simulink model "Suspension"  (R2019b)
settings: Solver=VariableStepAuto  StartTime=0.0  StopTime=10.0  RelTol=1e-3
values from neighbouring files (symbols this model uses):
  cfs = 1290    [Suspension_parameter.m]
  cft = 1000    [Suspension_parameter.m]
  crs = 1620    [Suspension_parameter.m]
  crt = 1000    [Suspension_parameter.m]
  iyy = 2460    [Suspension_parameter.m]
  kfs = 19960    [Suspension_parameter.m]
  kft = 175500    [Suspension_parameter.m]
  krs = 17500    [Suspension_parameter.m]
  krt = 175500    [Suspension_parameter.m]
  lf = 2.3    [Suspension_parameter.m]
  lr = 2.3    [Suspension_parameter.m]
  mc = 700    [Suspension_parameter.m]
  mf = 40    [Suspension_parameter.m]
  mr = 35.5    [Suspension_parameter.m]
libraries: simulink x4
(part 2 of 2)

== system Suspension/Sky Hook/Front Displacement(Zf)/Road condition 2  ==
  Product : Product  Inputs=3
  Saturation : Saturate  LowerLimit=0
  Scope : Scope
  Signal Generator : SignalGenerator  Amplitude=0.15  Frequency=1.852
  Step : Step  SampleTime=1.08
  Step1 : Step  Before=1  After=0  SampleTime=4
  Out2 : Outport
  wires:
  Signal Generator/1 -> Product/1
  Product/1 -> Out2/1, Saturation/1
  Step/1 -> Product/2
  Step1/1 -> Product/3
  Saturation/1 -> Scope/1

== system Suspension/Sky Hook/Front Displacement(Zf)/Sky Hook_f ==
  Zc_dot : Inport
  Zf_dot : Inport  Port=2
  Add : Sum  Inputs=+-
  Constant : Constant  Value=2838
  Constant1 : Constant  Value=258
  If : If  IfExpression=u1 >= 0  ZeroCross=off
  Merge : Merge
  Product : Product
  Switch Case Action Subsystem : Subsystem  TreatAsAtomicUnit=on
  Switch Case Action Subsystem1 : Subsystem  TreatAsAtomicUnit=on
  Out1 : Outport
  wires:
  Constant1/1 -> Switch Case Action Subsystem1/1(In1)
  Zc_dot/1 -> Product/1, Add/1
  Switch Case Action Subsystem/1(Out1) -> Merge/1
  Switch Case Action Subsystem1/1(Out1) -> Merge/2
  Add/1 -> Product/2
  Product/1 -> If/1
  If/2 -> Switch Case Action Subsystem1/Action
  If/1 -> Switch Case Action Subsystem/Action
  Constant/1 -> Switch Case Action Subsystem/1(In1)
  Zf_dot/1 -> Add/2
  Merge/1 -> Out1/1

== system Suspension/Sky Hook/Rear Displacement(Zr)/Road conditiion 1 ==
  Gain : Gain
  Product : Product  Inputs=3
  Scope : Scope
  Signal Generator : SignalGenerator  Amplitude=0.15  Frequency=1.852  Units=rad/sec
  Step : Step  SampleTime=1.08
  Step1 : Step  Before=1  After=0  SampleTime=1.35
  Out1 : Outport
  wires:
  Gain/1 -> Out1/1
  Step1/1 -> Product/3
  Product/1 -> Gain/1, Scope/1
  Step/1 -> Product/2
  Signal Generator/1 -> Product/1

== system Suspension/Sky Hook/Rear Displacement(Zr)/Road condition 2  ==
  Product : Product  Inputs=3
  Saturation : Saturate  LowerLimit=0
  Scope : Scope
  Signal Generator : SignalGenerator  Amplitude=0.15  Frequency=1.852
  Step : Step  SampleTime=1.08
  Step1 : Step  Before=1  After=0  SampleTime=4
  Out2 : Outport
  wires:
  Signal Generator/1 -> Product/1
  Product/1 -> Out2/1, Saturation/1
  Step/1 -> Product/2
  Step1/1 -> Product/3
  Saturation/1 -> Scope/1

== system Suspension/Sky Hook/Rear Displacement(Zr)/Sky Hook_r1 ==
  Zc_dot : Inport
  Zr_dot : Inport  Port=2
  Add : Sum  Inputs=+-
  Constant : Constant  Value=2838
  Constant1 : Constant  Value=258
  If : If  IfExpression=u1 >= 0  ZeroCross=off
  Merge : Merge
  Product : Product
  Switch Case Action Subsystem : Subsystem  TreatAsAtomicUnit=on
  Switch Case Action Subsystem1 : Subsystem  TreatAsAtomicUnit=on
  Out1 : Outport
  wires:
  Constant1/1 -> Switch Case Action Subsystem1/1(In1)
  Zc_dot/1 -> Product/1, Add/1
  Switch Case Action Subsystem/1(Out1) -> Merge/1
  Switch Case Action Subsystem1/1(Out1) -> Merge/2
  Add/1 -> Product/2
  Product/1 -> If/1
  If/2 -> Switch Case Action Subsystem1/Action
  If/1 -> Switch Case Action Subsystem/Action
  Constant/1 -> Switch Case Action Subsystem/1(In1)
  Zr_dot/1 -> Add/2
  Merge/1 -> Out1/1

== system Suspension/Ground Hook/Body Displacement(Zc)/Ground_hook_f/Switch Case Action Subsystem ==
  1 : Inport
  Action Port : ActionPort  ActionPortLabel=if(u1 >= 0)
  Csa : Outport
  wires:
  1/1 -> Csa/1

== system Suspension/Ground Hook/Body Displacement(Zc)/Ground_hook_f/Switch Case Action Subsystem2 ==
  In1 : Inport
  Action Port : ActionPort  ActionPortLabel=else
  Out1 : Outport
  wires:
  In1/1 -> Out1/1

== system Suspension/Ground Hook/Body Displacement(Zc)/Ground_hook_r/Switch Case Action Subsystem ==
  1 : Inport
  Action Port : ActionPort  ActionPortLabel=if(u1 >= 0)
  Csa : Outport
  wires:
  1/1 -> Csa/1

== system Suspension/Ground Hook/Body Displacement(Zc)/Ground_hook_r/Switch Case Action Subsystem2 ==
  In1 : Inport
  Action Port : ActionPort  ActionPortLabel=else
  Out1 : Outport
  wires:
  In1/1 -> Out1/1

== system Suspension/Ground Hook/Front Displacement(Zf)/Ground_hook_f/Switch Case Action Subsystem ==
  1 : Inport
  Action Port : ActionPort  ActionPortLabel=if(u1 >= 0)
  Csa : Outport
  wires:
  1/1 -> Csa/1

== system Suspension/Ground Hook/Front Displacement(Zf)/Ground_hook_f/Switch Case Action Subsystem2 ==
  In1 : Inport
  Action Port : ActionPort  ActionPortLabel=else
  Out1 : Outport
  wires:
  In1/1 -> Out1/1

== system Suspension/Ground Hook/Rear Displacement(Zr)/Ground_hook_r/Switch Case Action Subsystem ==
  1 : Inport
  Action Port : ActionPort  ActionPortLabel=if(u1 >= 0)
  Csa : Outport
  wires:
  1/1 -> Csa/1

== system Suspension/Ground Hook/Rear Displacement(Zr)/Ground_hook_r/Switch Case Action Subsystem2 ==
  In1 : Inport
  Action Port : ActionPort  ActionPortLabel=else
  Out1 : Outport
  wires:
  In1/1 -> Out1/1

== system Suspension/Hybird Hook/Body Displacement(Zc)/HybridHook_f/GroundHook ==
  In1 : Inport
  In2 : Inport  Port=2
  Add5 : Sum  Inputs=+-
  Constant : Constant  Value=2838
  Constant1 : Constant  Value=258
  Gain9 : Gain  Gain=-1
  If : If  IfExpression=u1 >= 0  ZeroCross=off
  Merge : Merge
  Product : Product
  Switch Case Action Subsystem : Subsystem  TreatAsAtomicUnit=on
  Switch Case Action Subsystem2 : Subsystem  TreatAsAtomicUnit=on
  Out1 : Outport
  wires:
  Gain9/1 -> Product/2
  In2/1 -> Gain9/1, Add5/2
  Product/1 -> If/1
  If/2 -> Switch Case Action Subsystem2/Action
  Switch Case Action Subsystem/1(Csa) -> Merge/1
  Switch Case Action Subsystem2/1(Out1) -> Merge/2
  Constant1/1 -> Switch Case Action Subsystem2/1(In1)
  If/1 -> Switch Case Action Subsystem/Action
  In1/1 -> Add5/1
  Constant/1 -> Switch Case Action Subsystem/1(1)
  Add5/1 -> Product/1
  Merge/1 -> Out1/1

== system Suspension/Hybird Hook/Body Displacement(Zc)/HybridHook_f/SkyHook ==
  In1 : Inport
  In2 : Inport  Port=2
  Add : Sum  Inputs=+-
  Constant2 : Constant  Value=2838
  Constant3 : Constant  Value=258
  If1 : If  IfExpression=u1 >= 0  ZeroCross=off
  Merge1 : Merge
  Product1 : Product
  Switch Case Action Subsystem1 : Subsystem  TreatAsAtomicUnit=on
  Switch Case Action Subsystem3 : Subsystem  TreatAsAtomicUnit=on
  Out1 : Outport
  wires:
  Product1/1 -> If1/1
  Constant2/1 -> Switch Case Action Subsystem1/1(In1)
  If1/1 -> Switch Case Action Subsystem1/Action
  Add/1 -> Product1/2
  Switch Case Action Subsystem1/1(Out1) -> Merge1/1
  Constant3/1 -> Switch Case Action Subsystem3/1(In1)
  In1/1 -> Product1/1, Add/1
  If1/2 -> Switch Case Action Subsystem3/Action
  Switch Case Action Subsystem3/1(Out1) -> Merge1/2
  Merge1/1 -> Out1/1
  In2/1 -> Add/2

== system Suspension/Hybird Hook/Body Displacement(Zc)/HybridHook_r/GroundHook ==
  In1 : Inport
  In2 : Inport  Port=2
  Add5 : Sum  Inputs=+-
  Constant : Constant  Value=2838
  Constant1 : Constant  Value=258
  Gain9 : Gain  Gain=-1
  If : If  IfExpression=u1 >= 0  ZeroCross=off
  Merge : Merge
  Product : Product
  Switch Case Action Subsystem : Subsystem  TreatAsAtomicUnit=on
  Switch Case Action Subsystem2 : Subsystem  TreatAsAtomicUnit=on
  Out1 : Outport
  wires:
  Gain9/1 -> Product/2
  In2/1 -> Gain9/1, Add5/2
  Product/1 -> If/1
  If/2 -> Switch Case Action Subsystem2/Action
  Switch Case Action Subsystem/1(Csa) -> Merge/1
  Switch Case Action Subsystem2/1(Out1) -> Merge/2
  Constant1/1 -> Switch Case Action Subsystem2/1(In1)
  If/1 -> Switch Case Action Subsystem/Action
  In1/1 -> Add5/1
  Constant/1 -> Switch Case Action Subsystem/1(1)
  Add5/1 -> Product/1
  Merge/1 -> Out1/1

== system Suspension/Hybird Hook/Body Displacement(Zc)/HybridHook_r/SkyHook ==
  In1 : Inport
  In2 : Inport  Port=2
  Add : Sum  Inputs=+-
  Constant2 : Constant  Value=2838
  Constant3 : Constant  Value=258
  If1 : If  IfExpression=u1 >= 0  ZeroCross=off
  Merge1 : Merge
  Product1 : Product
  Switch Case Action Subsystem1 : Subsystem  TreatAsAtomicUnit=on
  Switch Case Action Subsystem3 : Subsystem  TreatAsAtomicUnit=on
  Out1 : Outport
  wires:
  Product1/1 -> If1/1
  Constant2/1 -> Switch Case Action Subsystem1/1(In1)
  If1/1 -> Switch Case Action Subsystem1/Action
  Add/1 -> Product1/2
  Switch Case Action Subsystem1/1(Out1) -> Merge1/1
  Constant3/1 -> Switch Case Action Subsystem3/1(In1)
  In1/1 -> Product1/1, Add/1
  If1/2 -> Switch Case Action Subsystem3/Action
  Switch Case Action Subsystem3/1(Out1) -> Merge1/2
  Merge1/1 -> Out1/1
  In2/1 -> Add/2

== system Suspension/Hybird Hook/Front Displacement(Zf)/HybridHook_f/GroundHook ==
  In1 : Inport
  In2 : Inport  Port=2
  Add5 : Sum  Inputs=+-
  Constant : Constant  Value=2838
  Constant1 : Constant  Value=258
  Gain9 : Gain  Gain=-1
  If : If  IfExpression=u1 >= 0  ZeroCross=off
  Merge : Merge
  Product : Product
  Switch Case Action Subsystem : Subsystem  TreatAsAtomicUnit=on
  Switch Case Action Subsystem2 : Subsystem  TreatAsAtomicUnit=on
  Out1 : Outport
  wires:
  Gain9/1 -> Product/2
  In2/1 -> Gain9/1, Add5/2
  Product/1 -> If/1
  If/2 -> Switch Case Action Subsystem2/Action
  Switch Case Action Subsystem/1(Csa) -> Merge/1
  Switch Case Action Subsystem2/1(Out1) -> Merge/2
  Constant1/1 -> Switch Case Action Subsystem2/1(In1)
  If/1 -> Switch Case Action Subsystem/Action
  In1/1 -> Add5/1
  Constant/1 -> Switch Case Action Subsystem/1(1)
  Add5/1 -> Product/1
  Merge/1 -> Out1/1

== system Suspension/Hybird Hook/Front Displacement(Zf)/HybridHook_f/SkyHook ==
  In1 : Inport
  In2 : Inport  Port=2
  Add : Sum  Inputs=+-
  Constant2 : Constant  Value=2838
  Constant3 : Constant  Value=258
  If1 : If  IfExpression=u1 >= 0  ZeroCross=off
  Merge1 : Merge
  Product1 : Product
  Switch Case Action Subsystem1 : Subsystem  TreatAsAtomicUnit=on
  Switch Case Action Subsystem3 : Subsystem  TreatAsAtomicUnit=on
  Out1 : Outport
  wires:
  Product1/1 -> If1/1
  Constant2/1 -> Switch Case Action Subsystem1/1(In1)
  If1/1 -> Switch Case Action Subsystem1/Action
  Add/1 -> Product1/2
  Switch Case Action Subsystem1/1(Out1) -> Merge1/1
  Constant3/1 -> Switch Case Action Subsystem3/1(In1)
  In1/1 -> Product1/1, Add/1
  If1/2 -> Switch Case Action Subsystem3/Action
  Switch Case Action Subsystem3/1(Out1) -> Merge1/2
  Merge1/1 -> Out1/1
  In2/1 -> Add/2

== system Suspension/Hybird Hook/Rear Displacement(Zr)/HybridHook_r1/GroundHook ==
  In1 : Inport
  In2 : Inport  Port=2
  Add5 : Sum  Inputs=+-
  Constant : Constant  Value=2838
  Constant1 : Constant  Value=258
  Gain9 : Gain  Gain=-1
  If : If  IfExpression=u1 >= 0  ZeroCross=off
  Merge : Merge
  Product : Product
  Switch Case Action Subsystem : Subsystem  TreatAsAtomicUnit=on
  Switch Case Action Subsystem2 : Subsystem  TreatAsAtomicUnit=on
  Out1 : Outport
  wires:
  Gain9/1 -> Product/2
  In2/1 -> Gain9/1, Add5/2
  Product/1 -> If/1
  If/2 -> Switch Case Action Subsystem2/Action
  Switch Case Action Subsystem/1(Csa) -> Merge/1
  Switch Case Action Subsystem2/1(Out1) -> Merge/2
  Constant1/1 -> Switch Case Action Subsystem2/1(In1)
  If/1 -> Switch Case Action Subsystem/Action
  In1/1 -> Add5/1
  Constant/1 -> Switch Case Action Subsystem/1(1)
  Add5/1 -> Product/1
  Merge/1 -> Out1/1

== system Suspension/Hybird Hook/Rear Displacement(Zr)/HybridHook_r1/SkyHook ==
  In1 : Inport
  In2 : Inport  Port=2
  Add : Sum  Inputs=+-
  Constant2 : Constant  Value=2838
  Constant3 : Constant  Value=258
  If1 : If  IfExpression=u1 >= 0  ZeroCross=off
  Merge1 : Merge
  Product1 : Product
  Switch Case Action Subsystem1 : Subsystem  TreatAsAtomicUnit=on
  Switch Case Action Subsystem3 : Subsystem  TreatAsAtomicUnit=on
  Out1 : Outport
  wires:
  Product1/1 -> If1/1
  Constant2/1 -> Switch Case Action Subsystem1/1(In1)
  If1/1 -> Switch Case Action Subsystem1/Action
  Add/1 -> Product1/2
  Switch Case Action Subsystem1/1(Out1) -> Merge1/1
  Constant3/1 -> Switch Case Action Subsystem3/1(In1)
  In1/1 -> Product1/1, Add/1
  If1/2 -> Switch Case Action Subsystem3/Action
  Switch Case Action Subsystem3/1(Out1) -> Merge1/2
  Merge1/1 -> Out1/1
  In2/1 -> Add/2

== system Suspension/Sky Hook/Body Displacement(Zc)/Sky Hook_f/Switch Case Action Subsystem ==
  In1 : Inport
  Action Port : ActionPort  ActionPortLabel=if(u1 >= 0)
  Out1 : Outport
  wires:
  In1/1 -> Out1/1

== system Suspension/Sky Hook/Body Displacement(Zc)/Sky Hook_f/Switch Case Action Subsystem1 ==
  In1 : Inport
  Action Port : ActionPort  ActionPortLabel=else
  Out1 : Outport
  wires:
  In1/1 -> Out1/1

== system Suspension/Sky Hook/Body Displacement(Zc)/Sky Hook_r/Switch Case Action Subsystem ==
  In1 : Inport
  Action Port : ActionPort  ActionPortLabel=if(u1 >= 0)
  Out1 : Outport
  wires:
  In1/1 -> Out1/1

== system Suspension/Sky Hook/Body Displacement(Zc)/Sky Hook_r/Switch Case Action Subsystem1 ==
  In1 : Inport
  Action Port : ActionPort  ActionPortLabel=else
  Out1 : Outport
  wires:
  In1/1 -> Out1/1

== system Suspension/Sky Hook/Front Displacement(Zf)/Sky Hook_f/Switch Case Action Subsystem ==
  In1 : Inport
  Action Port : ActionPort  ActionPortLabel=if(u1 >= 0)
  Out1 : Outport
  wires:
  In1/1 -> Out1/1

== system Suspension/Sky Hook/Front Displacement(Zf)/Sky Hook_f/Switch Case Action Subsystem1 ==
  In1 : Inport
  Action Port : ActionPort  ActionPortLabel=else
  Out1 : Outport
  wires:
  In1/1 -> Out1/1

== system Suspension/Sky Hook/Rear Displacement(Zr)/Sky Hook_r1/Switch Case Action Subsystem ==
  In1 : Inport
  Action Port : ActionPort  ActionPortLabel=if(u1 >= 0)
  Out1 : Outport
  wires:
  In1/1 -> Out1/1

== system Suspension/Sky Hook/Rear Displacement(Zr)/Sky Hook_r1/Switch Case Action Subsystem1 ==
  In1 : Inport
  Action Port : ActionPort  ActionPortLabel=else
  Out1 : Outport
  wires:
  In1/1 -> Out1/1

== system Suspension/Hybird Hook/Body Displacement(Zc)/HybridHook_f/GroundHook/Switch Case Action Subsystem ==
  1 : Inport
  Action Port : ActionPort  ActionPortLabel=if(u1 >= 0)
  Csa : Outport
  wires:
  1/1 -> Csa/1

== system Suspension/Hybird Hook/Body Displacement(Zc)/HybridHook_f/GroundHook/Switch Case Action Subsystem2 ==
  In1 : Inport
  Action Port : ActionPort  ActionPortLabel=else
  Out1 : Outport
  wires:
  In1/1 -> Out1/1

== system Suspension/Hybird Hook/Body Displacement(Zc)/HybridHook_f/SkyHook/Switch Case Action Subsystem1 ==
  In1 : Inport
  Action Port : ActionPort  ActionPortLabel=if(u1 >= 0)
  Out1 : Outport
  wires:
  In1/1 -> Out1/1

== system Suspension/Hybird Hook/Body Displacement(Zc)/HybridHook_f/SkyHook/Switch Case Action Subsystem3 ==
  In1 : Inport
  Action Port : ActionPort  ActionPortLabel=else
  Out1 : Outport
  wires:
  In1/1 -> Out1/1

== system Suspension/Hybird Hook/Body Displacement(Zc)/HybridHook_r/GroundHook/Switch Case Action Subsystem ==
  1 : Inport
  Action Port : ActionPort  ActionPortLabel=if(u1 >= 0)
  Csa : Outport
  wires:
  1/1 -> Csa/1

== system Suspension/Hybird Hook/Body Displacement(Zc)/HybridHook_r/GroundHook/Switch Case Action Subsystem2 ==
  In1 : Inport
  Action Port : ActionPort  ActionPortLabel=else
  Out1 : Outport
  wires:
  In1/1 -> Out1/1

== system Suspension/Hybird Hook/Body Displacement(Zc)/HybridHook_r/SkyHook/Switch Case Action Subsystem1 ==
  In1 : Inport
  Action Port : ActionPort  ActionPortLabel=if(u1 >= 0)
  Out1 : Outport
  wires:
  In1/1 -> Out1/1

== system Suspension/Hybird Hook/Body Displacement(Zc)/HybridHook_r/SkyHook/Switch Case Action Subsystem3 ==
  In1 : Inport
  Action Port : ActionPort  ActionPortLabel=else
  Out1 : Outport
  wires:
  In1/1 -> Out1/1

== system Suspension/Hybird Hook/Front Displacement(Zf)/HybridHook_f/GroundHook/Switch Case Action Subsystem ==
  1 : Inport
  Action Port : ActionPort  ActionPortLabel=if(u1 >= 0)
  Csa : Outport
  wires:
  1/1 -> Csa/1

== system Suspension/Hybird Hook/Front Displacement(Zf)/HybridHook_f/GroundHook/Switch Case Action Subsystem2 ==
  In1 : Inport
  Action Port : ActionPort  ActionPortLabel=else
  Out1 : Outport
  wires:
  In1/1 -> Out1/1

== system Suspension/Hybird Hook/Front Displacement(Zf)/HybridHook_f/SkyHook/Switch Case Action Subsystem1 ==
  In1 : Inport
  Action Port : ActionPort  ActionPortLabel=if(u1 >= 0)
  Out1 : Outport
  wires:
  In1/1 -> Out1/1

== system Suspension/Hybird Hook/Front Displacement(Zf)/HybridHook_f/SkyHook/Switch Case Action Subsystem3 ==
  In1 : Inport
  Action Port : ActionPort  ActionPortLabel=else
  Out1 : Outport
  wires:
  In1/1 -> Out1/1

== system Suspension/Hybird Hook/Rear Displacement(Zr)/HybridHook_r1/GroundHook/Switch Case Action Subsystem ==
  1 : Inport
  Action Port : ActionPort  ActionPortLabel=if(u1 >= 0)
  Csa : Outport
  wires:
  1/1 -> Csa/1

== system Suspension/Hybird Hook/Rear Displacement(Zr)/HybridHook_r1/GroundHook/Switch Case Action Subsystem2 ==
  In1 : Inport
  Action Port : ActionPort  ActionPortLabel=else
  Out1 : Outport
  wires:
  In1/1 -> Out1/1

== system Suspension/Hybird Hook/Rear Displacement(Zr)/HybridHook_r1/SkyHook/Switch Case Action Subsystem1 ==
  In1 : Inport
  Action Port : ActionPort  ActionPortLabel=if(u1 >= 0)
  Out1 : Outport
  wires:
  In1/1 -> Out1/1

== system Suspension/Hybird Hook/Rear Displacement(Zr)/HybridHook_r1/SkyHook/Switch Case Action Subsystem3 ==
  In1 : Inport
  Action Port : ActionPort  ActionPortLabel=else
  Out1 : Outport
  wires:
  In1/1 -> Out1/1
